simulink library "ddm"  (R2021b)
settings: Solver=VariableStepAuto  StartTime=0.0  StopTime=10.0  RelTol=1e-3
undefined symbols (not defined in the file or in its folder): ADDM_FrTMTqDev_X_Nm, ADDM_RrTMTqDev_X_Nm, ENUM_ADASACCSTA_ERROR, ENUM_ADASACCSTA_OFF, ENUM_ADASACCSTA_STANDBY, ENUM_ALLOWMOV_ALLOWREADY, ENUM_APS, ENUM_BRKSTA_ERROR, ENUM_BRKSTA_OFF, ENUM_BRKSTA_ON, ENUM_BRKSW_INVALID, ENUM_BRKSW_OFF, ENUM_BRKSW_ON, ENUM_CHGPREACTERRSTA_OBCPRE, ENUM_DCDCFAULTSTA_ANYFAULTLV1, ENUM_DCDCFAULTSTA_ANYFAULTLV2, ENUM_DRIVETRAIN_AWD, ENUM_DRIVETRAIN_FWD, ENUM_DRIVETRAIN_RWD, ENUM_EDUDRTSTA_NORMAL, ENUM_EPBSTA_APPLIED, ENUM_EPBSTA_RELEASED, ENUM_GEARACTUALPOSN_INVALID, ENUM_GEARACTUALPOSN_P, ENUM_HVBATTREADYPRE_READY, ENUM_MCUWARN_LV0, ENUM_MCUWARN_LV1, ENUM_MCUWARN_LV2, ENUM_MCUWARN_LV3, ENUM_MCUWARN_NOERROR, ENUM_OBCFAULTSTA_ANYFAULT, ENUM_PAS_R2F2, ENUM_PDFAULT_BATTPDFAIL, ENUM_PDFAULT_DCDCDISABLE, ENUM_PDFAULT_MCUDISABLE, ENUM_PDFAULT_MCUDISCHRG, ENUM_POWERSTA_OFF, ENUM_POWERSTA_ON, ENUM_POWERSTA_READY, ENUM_POWERSTA_STANDBY, ENUM_PRESSINDI_LOW, ENUM_PUFAULT_BATTUPFAIL, ENUM_PUFAULT_DCDCENABLEFAIL, ENUM_PUFAULT_PRECHRGCHKFAIL, ENUM_PUFAULT_SAFETYCHKFAIL, ENUM_PUSTATE_COMPLETED, ENUM_PWRSTASW_OFF, ENUM_PWRSTASW_OFFA, ENUM_PWRSTASW_OFFCHVCHRG, ENUM_PWRSTASW_OFFCLVCHRG, ENUM_PWRSTASW_ON, ENUM_PWRSTASW_ONHVCHRG, ENUM_PWRSTASW_READY, ENUM_PWRSTASW_STANDBY, ENUM_SHIFTCOMMAND_P, ENUM_SHIFTERERRSTA_PBUTTONFAILURE, ENUM_VEHMALFUNLV_2ND, ENUM_VEHMALFUNLV_3RD, ENUM_VEHMALFUNLV_4TH, ENUM_VEHMALFUNLV_NORMAL ... (+459)
libraries: hcu_lib x521, $bdroot x5, simulink x3
(part 15 of 25)

== system ddm/DDM/DDM/TQD/Shifter1_DDM ==
  note: Release Condition After Decision
  note: Diagnostics and Fault Handling
  note: Diagnostics and Fault Handling
  note: Release Condition After Decision
  note: Release Condition After Decision
  note: Diagnostics and Fault Handling
  note: Shifter1 Rolling Count Error (Shifter1CSErr)
  note: Shifter1 Rolling Count Error (Shifter1RCErr)
  note: Shifter1 Lost Comm (Shifter1NoCom)
  task_time_s : Inport
  VPMM_SysPwrSta_enum : Inport  Port=2
  No_CAN3_BUS_OFF : Inport  Port=3
  VDDM_Shifter1NoCom_flg : Inport  Port=4
  VDDM_Shifter1RCErr_flg : Inport  Port=5
  VDDM_Shifter1CSErr_flg : Inport  Port=6
  DTC_clear_request : Inport  Port=7
  VINP_ShifterHandleCmd_enum : Inport  Port=8
  Constant1 : Constant  Value=KDDM_Shifter1NoComDTC_cnt
  Constant10 : Constant  Value=KDDM_Shifter1CSErrDTC_cnt
  Constant{3,11,16..17,19,24,31,36,48} (9 alike) : Constant  Value=ENUM_PWRSTASW_OFF
  Constant12 : Constant  Value=FALSE
  Constant13 : Constant  Value=KDDM_Shifter1RCErrDTC_cnt
  Constant14 : Constant  Value=KDDM_Shifter1RCErrPassTO_s
  Constant15 : Constant  Value=ZERO_INT
  Constant18 : Constant  Value=KDDM_Shifter1RCErrDetTO_s
  Constant2 : Constant  Value=FALSE
  Constant20 : Constant  Value=KDDM_Shifter1NoComDTC_cnt
  Constant21 : Constant  Value=KDDM_Shifter1NoComPassTO_s
  Constant22 : Constant  Value=KDDM_Shifter1NoComDetTO_s
  Constant23 : Constant  Value=ENUM_SHIFTCOMMAND_P
  Constant25 : Constant  Value=KDDM_TQDDiagnosisOffSW_flg
  Constant26 : Constant  Value=ENUM_PWRSTASW_STANDBY
  Constant27 : Constant  Value=KDDM_Shifter1RCErrPassTO_s
  Constant32 : Constant  Value=FALSE
  Constant33 : Constant  Value=KDDM_Shifter1CSErrDTC_cnt
  Constant34 : Constant  Value=KDDM_Shifter1CSErrPassTO_s
  Constant35 : Constant  Value=KDDM_Shifter1CSErrDetTO_s
  Constant4 : Constant  Value=KDDM_Shifter1RCErrDTC_cnt
  Constant41 : Constant  Value=KDDM_Shifter1CSErrPassTO_s
  Constant42 : Constant  Value=ENUM_SHIFTCOMMAND_P
  Constant44 : Constant  Value=KDDM_TQDDiagnosisOffSW_flg
  Constant45 : Constant  Value=ZERO_INT
  Constant5 : Constant  Value=ENUM_SHIFTCOMMAND_P
  Constant6 : Constant  Value=ENUM_PWRSTASW_STANDBY
  Constant7 : Constant  Value=KDDM_TQDDiagnosisOffSW_flg
  Constant70 : Constant  Value=KDDM_Shifter1NoComPassTO_s
  Constant8 : Constant  Value=ZERO_INT
  Constant9 : Constant  Value=ENUM_PWRSTASW_STANDBY
  DTC_Couter1 : hcu_lib/Basic_Blocks/DTC_Couter
  DTC_Couter2 : hcu_lib/Basic_Blocks/DTC_Couter
  DTC_Couter4 : hcu_lib/Basic_Blocks/DTC_Couter
  DTC_Info : hcu_lib/Basic_Blocks/DTC_Info
  DTC_Info1 : hcu_lib/Basic_Blocks/DTC_Info
  DTC_Info2 : hcu_lib/Basic_Blocks/DTC_Info
  Equal{,1,3,10..11,16..19} (9 alike) : RelationalOperator  Operator===  OutDataTypeStr=boolean  RndMeth=Simplest
  Equal{2,4..6,13..14} (6 alike) : RelationalOperator  Operator=~=  OutDataTypeStr=boolean  RndMeth=Simplest
  Equal15 : RelationalOperator  OutDataTypeStr=boolean  RndMeth=Simplest
  Equal7 : RelationalOperator  OutDataTypeStr=boolean  RndMeth=Simplest
  Equal8 : RelationalOperator  OutDataTypeStr=boolean  RndMeth=Simplest
  Logical Operator : Logic  Operator=OR  Inputs=3  AllPortsSameDT=off  OutDataTypeStr=boolean
  Logical Operator1 : Logic  Operator=OR  Inputs=4  AllPortsSameDT=off  OutDataTypeStr=boolean
  Logical Operator10 : Logic  Inputs=3  AllPortsSameDT=off  OutDataTypeStr=boolean
  Logical Operator{2,5,8,11,50..51} (6 alike) : Logic  AllPortsSameDT=off  OutDataTypeStr=boolean
  Logical Operator{6,9,12,14,20,24,28,30,34,38} (10 alike) : Logic  Operator=NOT  AllPortsSameDT=off  OutDataTypeStr=boolean
  Logical Operator{4,22,26,36} (4 alike) : Logic  Inputs=4  AllPortsSameDT=off  OutDataTypeStr=boolean
  Logical Operator3 : Logic  Operator=OR  Inputs=4  AllPortsSameDT=off  OutDataTypeStr=boolean
  Logical Operator48 : Logic  Operator=OR  Inputs=4  AllPortsSameDT=off  OutDataTypeStr=boolean
  Logical Operator7 : Logic  Inputs=3  AllPortsSameDT=off  OutDataTypeStr=boolean
  Relational Operator1 : RelationalOperator  Operator=>  OutDataTypeStr=boolean  RndMeth=Simplest
  Relational Operator2 : RelationalOperator  Operator=>  OutDataTypeStr=boolean  RndMeth=Simplest
  Relational Operator3 : RelationalOperator  Operator=>  OutDataTypeStr=boolean  RndMeth=Simplest
  Switch1 : Switch  Criteria=u2 ~= 0
  Switch2 : Switch  Criteria=u2 ~= 0
  Switch6 : Switch  Criteria=u2 ~= 0
  Terminator : Terminator
  Terminator1 : Terminator
  Terminator2 : Terminator
  Test Detection Criteria1 : hcu_lib/Basic_Blocks/Test Detection Criteria
  Test Detection Criteria2 : hcu_lib/Basic_Blocks/Test Detection Criteria
  Test Detection Criteria3 : hcu_lib/Basic_Blocks/Test Detection Criteria
  Timer1 : hcu_lib/Basic_Blocks/Timer
  Timer2 : hcu_lib/Basic_Blocks/Timer
  Timer3 : hcu_lib/Basic_Blocks/Timer
  Unit Delay1 : UnitDelay  SampleTime=-1  HasFrameUpgradeWarning=on
  Unit Delay2 : UnitDelay  SampleTime=-1  HasFrameUpgradeWarning=on
  Unit Delay6 : UnitDelay  SampleTime=-1  HasFrameUpgradeWarning=on
  VDDM_Shifter1NoComDTC_raw32 : Outport
  VDDM_Shifter1RCErrDTC_raw32 : Outport  Port=2
  VDDM_Shifter1CSErrDTC_raw32 : Outport  Port=3
  VDDM_Shifter1NoComCFS_flg : Outport  Port=4
  VDDM_Shifter1RCErrCFS_flg : Outport  Port=5
  VDDM_Shifter1CSErrCFS_flg : Outport  Port=6
  VDDM_Shifter1Err_flg : Outport  Port=7
  wires:
  [VPMM_SysPwrSta_enum] -> Equal3/1
  DTC_Couter2/2 -> Relational Operator3/1  "VDDM_Shifter1CSErrDTC_cnt"
  Equal1/1 -> Logical Operator5/2
  [VINP_ShifterHandleCmd_enum] -> Equal1/1
  Logical Operator3/1 -> [VDDM_Shifter1CSErrCFSRls_flg]  "VDDM_Shifter1CSErrCFSRls_flg"
  Constant23/1 -> Equal1/2
  Constant24/1 -> Equal19/2
  Constant8/1 -> Relational Operator3/2
  Logical Operator5/1 -> Logical Operator3/3
  Equal19/1 -> Logical Operator8/1
  Unit Delay1/1 -> Equal19/1
  Constant25/1 -> Logical Operator3/4
  [VDDM_Shifter1CSErrPass_flg] -> Logical Operator5/1
  [VDDM_Shifter1CSErrDet_flg] -> DTC_Couter2/1
  DTC_Couter2/1 -> [VDDM_Shifter1CSErrCFS_flg]  "VDDM_Shifter1CSErrCFS_flg"
  Constant10/1 -> DTC_Couter2/3
  [VDDM_Shifter1CSErrCFSRls_flg] -> DTC_Couter2/2
  [DTC_clear_request] -> Logical Operator3/2
  Relational Operator3/1 -> Terminator2/1  "VDDM_Shifter1CSErrDFS_flg"
  Constant9/1 -> Equal3/2
  Logical Operator8/1 -> Logical Operator3/1
  [VPMM_SysPwrSta_enum] -> Unit Delay1/1
  Equal3/1 -> Logical Operator8/2
  Equal11/1 -> Logical Operator2/2
  DTC_Couter1/1 -> [VDDM_Shifter1RCErrCFS_flg]  "VDDM_Shifter1RCErrCFS_flg"
  [DTC_clear_request] -> Logical Operator1/2
  Logical Operator2/1 -> Logical Operator1/1
  [VPMM_SysPwrSta_enum] -> Unit Delay2/1
  Constant6/1 -> Equal11/2
  Relational Operator1/1 -> Terminator1/1  "VDDM_Shifter1RCErrDFS_flg"
  DTC_Couter1/2 -> Relational Operator1/1  "VDDM_Shifter1RCErrDTC_cnt"
  [VDDM_Shifter1RCErrCFSRls_flg] -> DTC_Couter1/2
  [VINP_ShifterHandleCmd_enum] -> Equal10/1
  Constant5/1 -> Equal10/2
  Equal10/1 -> Logical Operator11/2
  [VDDM_Shifter1RCErrPass_flg] -> Logical Operator11/1
  [VDDM_Shifter1RCErrDet_flg] -> DTC_Couter1/1
  Logical Operator11/1 -> Logical Operator1/3
  Constant15/1 -> Relational Operator1/2
  [VPMM_SysPwrSta_enum] -> Equal11/1
  Equal16/1 -> Logical Operator2/1
  Constant7/1 -> Logical Operator1/4
  Logical Operator1/1 -> [VDDM_Shifter1RCErrCFSRls_flg]  "VDDM_Shifter1RCErrCFSRls_flg"
  Constant16/1 -> Equal16/2
  Unit Delay2/1 -> Equal16/1
  Constant4/1 -> DTC_Couter1/3
  Equal/1 -> Logical Operator51/2
  Constant42/1 -> Equal/2
  [VINP_ShifterHandleCmd_enum] -> Equal/1
  VINP_ShifterHandleCmd_enum/1 -> [VINP_ShifterHandleCmd_enum]
  Constant48/1 -> Equal18/2
  Unit Delay6/1 -> Equal18/1
  DTC_Couter4/2 -> Relational Operator2/1  "VDDM_Shifter1NoComDTC_cnt"
  [DTC_clear_request] -> Logical Operator48/2
  Constant26/1 -> Equal17/2
  Logical Operator50/1 -> Logical Operator48/1
  [VPMM_SysPwrSta_enum] -> Unit Delay6/1
  Equal17/1 -> Logical Operator50/2
  Relational Operator2/1 -> Terminator/1  "VDDM_Shifter1NoComDFS_flg"
  Constant44/1 -> Logical Operator48/4
  [VPMM_SysPwrSta_enum] -> Equal17/1
  Equal18/1 -> Logical Operator50/1
  Constant1/1 -> DTC_Couter4/3
  [VDDM_Shifter1NoComDet_flg] -> DTC_Couter4/1
  [VDDM_Shifter1NoComPass_flg] -> Logical Operator51/1
  Constant45/1 -> Relational Operator2/2
  Logical Operator51/1 -> Logical Operator48/3
  Logical Operator48/1 -> [VDDM_Shifter1NoComCFSRls_flg]  "VDDM_Shifter1NoComCFSRls_flg"
  [VDDM_Shifter1NoComCFSRls_flg] -> DTC_Couter4/2
  DTC_Couter4/1 -> [VDDM_Shifter1NoComCFS_flg]  "VDDM_Shifter1NoComCFS_flg"
  [VDDM_Shifter1CSErrCFS_flg] -> VDDM_Shifter1CSErrCFS_flg/1
  [VDDM_Shifter1RCErrCFS_flg] -> VDDM_Shifter1RCErrCFS_flg/1
  [VDDM_Shifter1NoComCFS_flg] -> VDDM_Shifter1NoComCFS_flg/1
  Logical Operator28/1 -> Logical Operator36/4
  [VDDM_Shifter1NoComCFS_flg] -> Logical Operator28/1
  Logical Operator6/1 -> Logical Operator22/4
  [VDDM_Shifter1NoComCFS_flg] -> Logical Operator6/1
  VDDM_Shifter1CSErr_flg/1 -> [VDDM_Shifter1CSErr_flg]
  VDDM_Shifter1RCErr_flg/1 -> [VDDM_Shifter1RCErr_flg]
  Switch2/1 -> Test Detection Criteria3/1
  Switch1/1 -> Test Detection Criteria2/1
  Test Detection Criteria3/1 -> [VDDM_Shifter1CSErrDet_flg]  "VDDM_Shifter1CSErrDet_flg"
  [VDDM_Shifter1CSErr_flg] -> Logical Operator26/3
  [DTC_clear_request] -> DTC_Info2/4
  Logical Operator38/1 -> Logical Operator36/3
  Logical Operator26/1 -> Switch2/3
  [VDDM_Shifter1CSErrCFS_flg] -> DTC_Info2/3
  Constant32/1 -> Switch2/1
  [VDDM_Shifter1CSErrCFSRls_flg] -> Switch2/2
  Timer3/1 -> Equal15/1
  Constant41/1 -> Timer3/4
  [task_time_s] -> Test Detection Criteria3/2
  [task_time_s] -> Timer3/3
  [VDDM_Shifter1CSErrDet_flg] -> DTC_Info2/1
  [No_CAN3_BUS_OFF] -> Logical Operator26/2
  [VPMM_SysPwrSta_enum] -> Equal14/1
  DTC_Info2/1 -> VDDM_Shifter1CSErrDTC_raw32/1  "VDDM_Shifter1CSErrDTC_raw32"
  Equal13/1 -> Logical Operator36/1
  [No_CAN3_BUS_OFF] -> Logical Operator36/2
  [VDDM_Shifter1CSErrPass_flg] -> DTC_Info2/2
  Constant35/1 -> Test Detection Criteria3/4
  Constant31/1 -> Equal14/2
  Constant36/1 -> Equal13/2
  [VDDM_Shifter1CSErr_flg] -> Logical Operator38/1
  Constant34/1 -> Equal15/2
  [VDDM_Shifter1NoComCFS_flg] -> Logical Operator34/1
  Logical Operator36/1 -> Logical Operator30/1, Timer3/1
  Equal14/1 -> Logical Operator26/1
  Equal15/1 -> [VDDM_Shifter1CSErrPass_flg]  "VDDM_Shifter1CSErrPass_flg"
  Constant33/1 -> Test Detection Criteria3/3
  [VPMM_SysPwrSta_enum] -> Equal13/1
  Logical Operator30/1 -> Timer3/2
  Logical Operator34/1 -> Logical Operator26/4
  Test Detection Criteria2/1 -> [VDDM_Shifter1RCErrDet_flg]  "VDDM_Shifter1RCErrDet_flg"
  [VDDM_Shifter1RCErr_flg] -> Logical Operator4/3
  [DTC_clear_request] -> DTC_Info1/4
  Logical Operator24/1 -> Logical Operator22/3
  Logical Operator4/1 -> Switch1/3
  [VDDM_Shifter1RCErrCFS_flg] -> DTC_Info1/3
  Constant12/1 -> Switch1/1
  [VDDM_Shifter1RCErrCFSRls_flg] -> Switch1/2
  Timer1/1 -> Equal8/1
  Constant27/1 -> Timer1/4
  [task_time_s] -> Test Detection Criteria2/2
  [task_time_s] -> Timer1/3
  [VDDM_Shifter1RCErrDet_flg] -> DTC_Info1/1
  [No_CAN3_BUS_OFF] -> Logical Operator4/2
  [VPMM_SysPwrSta_enum] -> Equal5/1
  DTC_Info1/1 -> VDDM_Shifter1RCErrDTC_raw32/1  "VDDM_Shifter1RCErrDTC_raw32"
  Equal4/1 -> Logical Operator22/1
  [No_CAN3_BUS_OFF] -> Logical Operator22/2
  [VDDM_Shifter1RCErrPass_flg] -> DTC_Info1/2
  Constant18/1 -> Test Detection Criteria2/4
  Constant11/1 -> Equal5/2
  Constant19/1 -> Equal4/2
  [VDDM_Shifter1RCErr_flg] -> Logical Operator24/1
  Constant14/1 -> Equal8/2
  [VDDM_Shifter1NoComCFS_flg] -> Logical Operator20/1
  Logical Operator22/1 -> Logical Operator12/1, Timer1/1
  Equal5/1 -> Logical Operator4/1
  Equal8/1 -> [VDDM_Shifter1RCErrPass_flg]  "VDDM_Shifter1RCErrPass_flg"
  Constant13/1 -> Test Detection Criteria2/3
  [VPMM_SysPwrSta_enum] -> Equal4/1
  Logical Operator12/1 -> Timer1/2
  Logical Operator20/1 -> Logical Operator4/4
  Constant2/1 -> Switch6/1
  Logical Operator10/1 -> Switch6/3
  Switch6/1 -> Test Detection Criteria1/1
  [VDDM_Shifter1NoComCFSRls_flg] -> Switch6/2
  [DTC_clear_request] -> DTC_Info/4
  No_CAN3_BUS_OFF/1 -> [No_CAN3_BUS_OFF]
  [VDDM_Shifter1NoComDet_flg] -> DTC_Info/1
  DTC_clear_request/1 -> [DTC_clear_request]
  task_time_s/1 -> [task_time_s]
  [VDDM_Shifter1NoComPass_flg] -> DTC_Info/2
  DTC_Info/1 -> VDDM_Shifter1NoComDTC_raw32/1  "VDDM_Shifter1NoComDTC_raw32"
  [VDDM_Shifter1NoComCFS_flg] -> DTC_Info/3
  VPMM_SysPwrSta_enum/1 -> [VPMM_SysPwrSta_enum]
  VDDM_Shifter1NoCom_flg/1 -> [VDDM_Shifter1NoCom_flg]
  [VPMM_SysPwrSta_enum] -> Equal2/1
  [No_CAN3_BUS_OFF] -> Logical Operator7/2
  Constant3/1 -> Equal2/2
  Logical Operator9/1 -> Logical Operator7/3
  Equal2/1 -> Logical Operator7/1
  [VDDM_Shifter1NoCom_flg] -> Logical Operator9/1
  [VPMM_SysPwrSta_enum] -> Equal6/1
  [VDDM_Shifter1NoCom_flg] -> Logical Operator10/3
  Constant17/1 -> Equal6/2
  Equal6/1 -> Logical Operator10/1
  [No_CAN3_BUS_OFF] -> Logical Operator10/2
  [task_time_s] -> Timer2/3
  Constant21/1 -> Equal7/2
  [task_time_s] -> Test Detection Criteria1/2
  Constant70/1 -> Timer2/4
  Constant20/1 -> Test Detection Criteria1/3
  Test Detection Criteria1/1 -> [VDDM_Shifter1NoComDet_flg]  "VDDM_Shifter1NoComDet_flg"
  Equal7/1 -> [VDDM_Shifter1NoComPass_flg]  "VDDM_Shifter1NoComPass_flg"
  Timer2/1 -> Equal7/1
  Logical Operator7/1 -> Timer2/1, Logical Operator14/1
  Constant22/1 -> Test Detection Criteria1/4
  Logical Operator14/1 -> Timer2/2
  [VDDM_Shifter1NoComCFS_flg] -> Logical Operator/1
  [VDDM_Shifter1RCErrCFS_flg] -> Logical Operator/2
  [VDDM_Shifter1CSErrCFS_flg] -> Logical Operator/3
  Logical Operator/1 -> VDDM_Shifter1Err_flg/1  "VDDM_Shifter1Err_flg"

== system ddm/DDM/DDM/VMC_DDM/ACC Acceleration Command Error ==
  task_time_s : Inport
  VDDM_FCM1NoComCFS_flg : Inport  Port=2
  VDDM_FCM1RCErrCFS_flg : Inport  Port=3
  VDDM_FCM1CSErrCFS_flg : Inport  Port=4
  VVMC_ADASActive_flg : Inport  Port=5
  No_CAN6_BUS_OFF : Inport  Port=6
  VPMM_PowerSta_enum : Inport  Port=7
  VINP_ACCRequireAccel_mps2 : Inport  Port=8
  VINP_ADASACCSta_enum : Inport  Port=9
  DTC_clear_request : Inport  Port=10
  "ACC Acceleration Command Error " : Subsystem
  VDDM_ACCAccelCmdErrCFS_flg : Outport
  VDDM_ACCAccelCmdErrDetDTC_raw32 : Outport  Port=2
  wires:
  [VDDM_ACCAccelCmdErrDetDTC_raw32] -> VDDM_ACCAccelCmdErrDetDTC_raw32/1
  "ACC Acceleration Command Error "/2(VDDM_ACCAccelCmdErrDetDTC_raw32) -> [VDDM_ACCAccelCmdErrDetDTC_raw32]
  VINP_ADASACCSta_enum/1 -> [VINP_ADASACCSta_enum]
  [VINP_ADASACCSta_enum] -> "ACC Acceleration Command Error "/9(VINP_ADASACCSta_enum)
  [VVMC_ADASActive_flg] -> "ACC Acceleration Command Error "/5(VVMC_ADASActive_flg)
  VVMC_ADASActive_flg/1 -> [VVMC_ADASActive_flg]
  [task_time_s] -> "ACC Acceleration Command Error "/1(task_time_s)
  task_time_s/1 -> [task_time_s]  "task_time_s"
  [DTC_clear_request] -> "ACC Acceleration Command Error "/10(DTC_clear_request)
  [VINP_ACCRequireAccel_mps2] -> "ACC Acceleration Command Error "/8(VINP_ACCRequireAccel_mps2)
  [VPMM_PowerSta_enum] -> "ACC Acceleration Command Error "/7(VPMM_PowerSta_enum)
  [No_CAN6_BUS_OFF] -> "ACC Acceleration Command Error "/6(No_CAN6_BUS_OFF)
  [VDDM_FCM1CSErrCFS_flg] -> "ACC Acceleration Command Error "/4(VDDM_FCM1CSErrCFS_flg)
  [VDDM_FCM1RCErrCFS_flg] -> "ACC Acceleration Command Error "/3(VDDM_FCM1RCErrCFS_flg)
  [VDDM_FCM1NoComCFS_flg] -> "ACC Acceleration Command Error "/2(VDDM_FCM1NoComCFS_flg)
  VINP_ACCRequireAccel_mps2/1 -> [VINP_ACCRequireAccel_mps2]
  VDDM_FCM1NoComCFS_flg/1 -> [VDDM_FCM1NoComCFS_flg]
  No_CAN6_BUS_OFF/1 -> [No_CAN6_BUS_OFF]
  VPMM_PowerSta_enum/1 -> [VPMM_PowerSta_enum]
  DTC_clear_request/1 -> [DTC_clear_request]
  "ACC Acceleration Command Error "/1(VDDM_ACCAccelCmdErrCFS_flg) -> [VDDM_ACCAccelCmdErrCFS_flg]
  [VDDM_ACCAccelCmdErrCFS_flg] -> VDDM_ACCAccelCmdErrCFS_flg/1
  VDDM_FCM1RCErrCFS_flg/1 -> [VDDM_FCM1RCErrCFS_flg]
  VDDM_FCM1CSErrCFS_flg/1 -> [VDDM_FCM1CSErrCFS_flg]

== system ddm/DDM/DDM/VMC_DDM/BMS Signal Error  ==
  task_time_s : Inport
  VDDM_C3BMS6LCCFS_flg : Inport  Port=2
  VDDM_C3BMS6RCCFS_flg : Inport  Port=3
  VDDM_C3BMS6CSCFS_flg : Inport  Port=4
  No_CAN3_BUS_OFF : Inport  Port=5
  VPMM_PowerSta_enum : Inport  Port=6
  VINP_BMSWarn8_flg : Inport  Port=7
  VINP_BMSWarn7_flg : Inport  Port=8
  VINP_BMSWarn6_flg : Inport  Port=9
  VINP_BMSWarn5_flg : Inport  Port=10
  VINP_BMSWarn4_flg : Inport  Port=11
  VINP_BMSWarn3_flg : Inport  Port=12
  VINP_BMSWarn2_flg : Inport  Port=13
  VINP_BMSWarn1_flg : Inport  Port=14
  DTC_clear_request : Inport  Port=15
  "BMS Signal Error " : Subsystem
  VDDM_BMSSigErrCFS_flg : Outport
  VDDM_BMSSigErrDetDTC_raw32 : Outport  Port=2
  wires:
  [VDDM_BMSSigErrDetDTC_raw32] -> VDDM_BMSSigErrDetDTC_raw32/1
  "BMS Signal Error "/2(VDDM_BMSSigErrDetDTC_raw32) -> [VDDM_BMSSigErrDetDTC_raw32]
  [task_time_s] -> "BMS Signal Error "/1(task_time_s)
  task_time_s/1 -> [task_time_s]  "task_time_s"
  [VINP_BMSWarn8_flg] -> "BMS Signal Error "/15(VINP_BMSWarn8_flg)
  [VPMM_PowerSta_enum] -> "BMS Signal Error "/6(VPMM_PowerSta_enum)
  [No_CAN3_BUS_OFF] -> "BMS Signal Error "/5(No_CAN3_BUS_OFF)
  [VDDM_C3BMS6RCCFS_flg] -> "BMS Signal Error "/3(VDDM_C3BMS6RCCFS_flg)
  [VDDM_C3BMS6LCCFS_flg] -> "BMS Signal Error "/2(VDDM_C3BMS6LCCFS_flg)
  VINP_BMSWarn4_flg/1 -> [VINP_BMSWarn4_flg]
  VINP_BMSWarn6_flg/1 -> [VINP_BMSWarn6_flg]
  VINP_BMSWarn5_flg/1 -> [VINP_BMSWarn5_flg]
  VINP_BMSWarn7_flg/1 -> [VINP_BMSWarn7_flg]
  VINP_BMSWarn8_flg/1 -> [VINP_BMSWarn8_flg]
  VDDM_C3BMS6LCCFS_flg/1 -> [VDDM_C3BMS6LCCFS_flg]
  No_CAN3_BUS_OFF/1 -> [No_CAN3_BUS_OFF]
  VPMM_PowerSta_enum/1 -> [VPMM_PowerSta_enum]
  DTC_clear_request/1 -> [DTC_clear_request]
  "BMS Signal Error "/1(VDDM_BMSSigErrCFS_flg) -> [VDDM_BMSSigErrCFS_flg]
  [VDDM_BMSSigErrCFS_flg] -> VDDM_BMSSigErrCFS_flg/1
  VDDM_C3BMS6RCCFS_flg/1 -> [VDDM_C3BMS6RCCFS_flg]
  VDDM_C3BMS6CSCFS_flg/1 -> [VDDM_C3BMS6CSCFS_flg]
  [VDDM_C3BMS6CSCFS_flg] -> "BMS Signal Error "/4(VDDM_C3BMS6CSCFS_flg)
  [DTC_clear_request] -> "BMS Signal Error "/10(DTC_clear_request)
  [VINP_BMSWarn5_flg] -> "BMS Signal Error "/12(VINP_BMSWarn5_flg)
  [VINP_BMSWarn4_flg] -> "BMS Signal Error "/11(VINP_BMSWarn4_flg)
  [VINP_BMSWarn6_flg] -> "BMS Signal Error "/13(VINP_BMSWarn6_flg)
  [VINP_BMSWarn7_flg] -> "BMS Signal Error "/14(VINP_BMSWarn7_flg)
  [VINP_BMSWarn1_flg] -> "BMS Signal Error "/7(VINP_BMSWarn1_flg)
  [VINP_BMSWarn2_flg] -> "BMS Signal Error "/8(VINP_BMSWarn2_flg)
  [VINP_BMSWarn3_flg] -> "BMS Signal Error "/9(VINP_BMSWarn3_flg)
  VINP_BMSWarn3_flg/1 -> [VINP_BMSWarn3_flg]
  VINP_BMSWarn2_flg/1 -> [VINP_BMSWarn2_flg]
  VINP_BMSWarn1_flg/1 -> [VINP_BMSWarn1_flg]

== system ddm/DDM/DDM/VMC_DDM/CCU Signal Error ==
  task_time_s : Inport
  VDDM_C3CCU2LCCFS_flg : Inport  Port=2
  VDDM_C3CCU2RCCFS_flg : Inport  Port=3
  VDDM_C3CCU2CSCFS_flg : Inport  Port=4
  No_CAN3_BUS_OFF : Inport  Port=5
  VPMM_PowerSta_enum : Inport  Port=6
  VINP_DCDCFaultSta_enum : Inport  Port=7
  DTC_clear_request : Inport  Port=8
  "CCU Signal Error " : Subsystem
  VDDM_CCUSigErrCFS_flg : Outport
  VDDM_CCUSigErrDetDTC_raw32 : Outport  Port=2
  wires:
  [VDDM_CCUSigErrDetDTC_raw32] -> VDDM_CCUSigErrDetDTC_raw32/1
  "CCU Signal Error "/2(VDDM_CCUSigErrDetDTC_raw32) -> [VDDM_CCUSigErrDetDTC_raw32]
  [task_time_s] -> "CCU Signal Error "/1(task_time_s)
  task_time_s/1 -> [task_time_s]  "task_time_s"
  [DTC_clear_request] -> "CCU Signal Error "/8(DTC_clear_request)
  [VINP_DCDCFaultSta_enum] -> "CCU Signal Error "/7(VINP_DCDCFaultSta_enum)
  [VPMM_PowerSta_enum] -> "CCU Signal Error "/6(VPMM_PowerSta_enum)
  [No_CAN3_BUS_OFF] -> "CCU Signal Error "/5(No_CAN3_BUS_OFF)
  [VDDM_C3CCU2CSCFS_flg] -> "CCU Signal Error "/4(VDDM_C3CCU2CSCFS_flg)
  [VDDM_C3CCU2RCCFS_flg] -> "CCU Signal Error "/3(VDDM_C3CCU2RCCFS_flg)
  [VDDM_C3CCU2LCCFS_flg] -> "CCU Signal Error "/2(VDDM_C3CCU2LCCFS_flg)
  VINP_DCDCFaultSta_enum/1 -> [VINP_DCDCFaultSta_enum]
  VDDM_C3CCU2LCCFS_flg/1 -> [VDDM_C3CCU2LCCFS_flg]
  No_CAN3_BUS_OFF/1 -> [No_CAN3_BUS_OFF]
  VPMM_PowerSta_enum/1 -> [VPMM_PowerSta_enum]
  DTC_clear_request/1 -> [DTC_clear_request]
  "CCU Signal Error "/1(VDDM_CCUSigErrCFS_flg) -> [VDDM_CCUSigErrCFS_flg]
  [VDDM_CCUSigErrCFS_flg] -> VDDM_CCUSigErrCFS_flg/1
  VDDM_C3CCU2RCCFS_flg/1 -> [VDDM_C3CCU2RCCFS_flg]
  VDDM_C3CCU2CSCFS_flg/1 -> [VDDM_C3CCU2CSCFS_flg]

== system ddm/DDM/DDM/VMC_DDM/ESC Signal Error ==
  task_time_s : Inport
  No_CAN1_BUS_OFF : Inport  Port=2
  VPMM_PowerSta_enum : Inport  Port=3
  DTC_clear_request : Inport  Port=4
  VDDM_ESC1NoComCFS_flg : Inport  Port=5
  VDDM_ESC1RCErrCFS_flg : Inport  Port=6
  VDDM_ESC1CSErrCFS_flg : Inport  Port=7
  VDDM_ESC5NoComCFS_flg : Inport  Port=8
  VDDM_ESC5RCErrCFS_flg : Inport  Port=9
  VDDM_ESC5CSErrCFS_flg : Inport  Port=10
  VINP_HDDFailed_flg : Inport  Port=11
  VINP_EBDFailed_flg : Inport  Port=12
  VINP_ABSFailed_flg : Inport  Port=13
  VINP_TCSFailed_flg : Inport  Port=14
  VINP_ESCFailed_flg : Inport  Port=15
  VINP_HBBFailed_flg : Inport  Port=16
  VINP_PBAFailed_flg : Inport  Port=17
  VINP_HSAFailed_flg : Inport  Port=18
  VINP_AVHFailed_flg : Inport  Port=19
  VINP_MCPressureV_flg : Inport  Port=20
  VINP_BrkSwV_flg : Inport  Port=21
  VINP_BrkPedalPosSta_flg : Inport  Port=22
  VINP_LongAccelV_flg : Inport  Port=23
  VINP_LatAccelV_flg : Inport  Port=24
  VINP_YawRateV_flg : Inport  Port=25
  VINP_RFPulseCountV_flg : Inport  Port=26
  VINP_RRPulseCountV_flg : Inport  Port=27
  VINP_LFPulseCountV_flg : Inport  Port=28
  VINP_LRPulseCountV_flg : Inport  Port=29
  VINP_LRRawWhlSpeedV_flg : Inport  Port=30
  VINP_RRRawWhlSpeedV_flg : Inport  Port=31
  VINP_LFRawWhlSpeedV_flg : Inport  Port=32
  VINP_RFRawWhlSpeedV_flg : Inport  Port=33
  "ESC Signal Error " : Subsystem
  VDDM_ESCSigErrCFS_flg : Outport
  VDDM_ESCSigErrDetDTC_raw32 : Outport  Port=2
  VDDM_ESC1SigErr_flg : Outport  Port=3
  VDDM_ESC5SigErr_flg : Outport  Port=4
  wires:
  [VDDM_ESC5SigErr_flg] -> VDDM_ESC5SigErr_flg/1
  [VDDM_ESC1SigErr_flg] -> VDDM_ESC1SigErr_flg/1
  "ESC Signal Error "/4(VDDM_ESC5SigErr_flg) -> [VDDM_ESC5SigErr_flg]
  "ESC Signal Error "/3(VDDM_ESC1SigErr_flg) -> [VDDM_ESC1SigErr_flg]
  [VINP_RFRawWhlSpeedV_flg] -> "ESC Signal Error "/33(VINP_RFRawWhlSpeedV_flg)
  [VINP_LFRawWhlSpeedV_flg] -> "ESC Signal Error "/32(VINP_LFRawWhlSpeedV_flg)
  [VINP_RRRawWhlSpeedV_flg] -> "ESC Signal Error "/31(VINP_RRRawWhlSpeedV_flg)
  [VINP_LRRawWhlSpeedV_flg] -> "ESC Signal Error "/30(VINP_LRRawWhlSpeedV_flg)
  [VINP_LRPulseCountV_flg] -> "ESC Signal Error "/29(VINP_LRPulseCountV_flg)
  [VINP_LFPulseCountV_flg] -> "ESC Signal Error "/28(VINP_LFPulseCountV_flg)
  [VINP_RRPulseCountV_flg] -> "ESC Signal Error "/27(VINP_RRPulseCountV_flg)
  [VINP_RFPulseCountV_flg] -> "ESC Signal Error "/26(VINP_RFPulseCountV_flg)
  VINP_RFRawWhlSpeedV_flg/1 -> [VINP_RFRawWhlSpeedV_flg]
  VINP_RRRawWhlSpeedV_flg/1 -> [VINP_RRRawWhlSpeedV_flg]
  VINP_LFRawWhlSpeedV_flg/1 -> [VINP_LFRawWhlSpeedV_flg]
  VINP_LRRawWhlSpeedV_flg/1 -> [VINP_LRRawWhlSpeedV_flg]
  VINP_LRPulseCountV_flg/1 -> [VINP_LRPulseCountV_flg]
  VINP_LFPulseCountV_flg/1 -> [VINP_LFPulseCountV_flg]
  VINP_RRPulseCountV_flg/1 -> [VINP_RRPulseCountV_flg]
  VINP_RFPulseCountV_flg/1 -> [VINP_RFPulseCountV_flg]
  [VDDM_ESCSigErrCFS_flg] -> VDDM_ESCSigErrCFS_flg/1
  [VINP_YawRateV_flg] -> "ESC Signal Error "/25(VINP_YawRateV_flg)
  [VINP_LatAccelV_flg] -> "ESC Signal Error "/24(VINP_LatAccelV_flg)
  [VINP_LongAccelV_flg] -> "ESC Signal Error "/23(VINP_LongAccelV_flg)
  [VINP_BrkPedalPosSta_flg] -> "ESC Signal Error "/22(VINP_BrkPedalPosSta_flg)
  [VINP_BrkSwV_flg] -> "ESC Signal Error "/21(VINP_BrkSwV_flg)
  [VINP_MCPressureV_flg] -> "ESC Signal Error "/20(VINP_MCPressureV_flg)
  [VINP_AVHFailed_flg] -> "ESC Signal Error "/19(VINP_AVHFailed_flg)
  [VINP_HSAFailed_flg] -> "ESC Signal Error "/18(VINP_HSAFailed_flg)
  [VINP_PBAFailed_flg] -> "ESC Signal Error "/17(VINP_PBAFailed_flg)
  [VINP_HBBFailed_flg] -> "ESC Signal Error "/16(VINP_HBBFailed_flg)
  [VINP_ESCFailed_flg] -> "ESC Signal Error "/15(VINP_ESCFailed_flg)
  [VINP_TCSFailed_flg] -> "ESC Signal Error "/14(VINP_TCSFailed_flg)
  [VINP_ABSFailed_flg] -> "ESC Signal Error "/13(VINP_ABSFailed_flg)
  [VINP_EBDFailed_flg] -> "ESC Signal Error "/12(VINP_EBDFailed_flg)
  [VINP_HDDFailed_flg] -> "ESC Signal Error "/11(VINP_HDDFailed_flg)
  VINP_YawRateV_flg/1 -> [VINP_YawRateV_flg]
  VINP_LatAccelV_flg/1 -> [VINP_LatAccelV_flg]
  VINP_LongAccelV_flg/1 -> [VINP_LongAccelV_flg]
  VINP_BrkPedalPosSta_flg/1 -> [VINP_BrkPedalPosSta_flg]
  VINP_BrkSwV_flg/1 -> [VINP_BrkSwV_flg]
  VINP_MCPressureV_flg/1 -> [VINP_MCPressureV_flg]
  VINP_AVHFailed_flg/1 -> [VINP_AVHFailed_flg]
  VINP_HSAFailed_flg/1 -> [VINP_HSAFailed_flg]
  VINP_PBAFailed_flg/1 -> [VINP_PBAFailed_flg]
  VINP_HBBFailed_flg/1 -> [VINP_HBBFailed_flg]
  VINP_ESCFailed_flg/1 -> [VINP_ESCFailed_flg]
  VINP_TCSFailed_flg/1 -> [VINP_TCSFailed_flg]
  VINP_ABSFailed_flg/1 -> [VINP_ABSFailed_flg]
  VINP_EBDFailed_flg/1 -> [VINP_EBDFailed_flg]
  VINP_HDDFailed_flg/1 -> [VINP_HDDFailed_flg]
  [VDDM_ESC5CSErrCFS_flg] -> "ESC Signal Error "/10(VDDM_ESC5CSErrCFS_flg)
  [VDDM_ESC5RCErrCFS_flg] -> "ESC Signal Error "/9(VDDM_ESC5RCErrCFS_flg)
  [VDDM_ESC5NoComCFS_flg] -> "ESC Signal Error "/8(VDDM_ESC5NoComCFS_flg)
  VDDM_ESC5NoComCFS_flg/1 -> [VDDM_ESC5NoComCFS_flg]
  VDDM_ESC5RCErrCFS_flg/1 -> [VDDM_ESC5RCErrCFS_flg]
  VDDM_ESC5CSErrCFS_flg/1 -> [VDDM_ESC5CSErrCFS_flg]
  "ESC Signal Error "/1(VDDM_ESCSigErrCFS_flg) -> [VDDM_ESCSigErrCFS_flg]
  DTC_clear_request/1 -> [DTC_clear_request]
  VPMM_PowerSta_enum/1 -> [VPMM_PowerSta_enum]
  No_CAN1_BUS_OFF/1 -> [No_CAN1_BUS_OFF]
  [No_CAN1_BUS_OFF] -> "ESC Signal Error "/2(No_CAN1_BUS_OFF)
  [VPMM_PowerSta_enum] -> "ESC Signal Error "/3(VPMM_PowerSta_enum)
  [DTC_clear_request] -> "ESC Signal Error "/4(DTC_clear_request)
  task_time_s/1 -> [task_time_s]  "task_time_s"
  [task_time_s] -> "ESC Signal Error "/1(task_time_s)
  "ESC Signal Error "/2(VDDM_ESCSigErrDetDTC_raw32) -> [VDDM_ESCSigErrDetDTC_raw32]
  [VDDM_ESCSigErrDetDTC_raw32] -> VDDM_ESCSigErrDetDTC_raw32/1
  VDDM_ESC1NoComCFS_flg/1 -> [VDDM_ESC1NoComCFS_flg]
  VDDM_ESC1RCErrCFS_flg/1 -> [VDDM_ESC1RCErrCFS_flg]
  VDDM_ESC1CSErrCFS_flg/1 -> [VDDM_ESC1CSErrCFS_flg]
  [VDDM_ESC1NoComCFS_flg] -> "ESC Signal Error "/5(VDDM_ESC1NoComCFS_flg)
  [VDDM_ESC1RCErrCFS_flg] -> "ESC Signal Error "/6(VDDM_ESC1RCErrCFS_flg)
  [VDDM_ESC1CSErrCFS_flg] -> "ESC Signal Error "/7(VDDM_ESC1CSErrCFS_flg)

== system ddm/DDM/DDM/VMC_DDM/Enabled Subsystem ==
  task_time_s : Inport
  VPMM_PowerSta_enum : Inport  Port=2
  VDDM_EPS1NoCom_flg : Inport  Port=3
  No_CAN1_BUS_OFF : Inport  Port=4
  DTC_clear_request : Inport  Port=5
  VTQD_GearActualPosn_enum : Inport  Port=6
  VDDM_EPSRCErr_flg : Inport  Port=7
  VDDM_EPSCSErr_flg : Inport  Port=8
  VINP_SASV_flg : Inport  Port=9
  EPS1 Checksum Error : Subsystem
  EPS1 Lost Comm : Subsystem
  "EPS1 Rolling Count Error " : Subsystem
  EPS1 Signal Error : Subsystem
  VDDM_EPS1NoComCFS_flg : Outport
  VDDM_EPS1NoComDTC_raw32 : Outport  Port=2
  VDDM_EPS1RCErrCFS_flg : Outport  Port=3
  VDDM_EPS1RCErrDTC_raw32 : Outport  Port=4
  VDDM_EPS1CSErrCFS_flg : Outport  Port=5
  VDDM_EPS1CSErrDTC_raw32 : Outport  Port=6
  VDDM_EPSSigErrCFS_flg : Outport  Port=7
  VDDM_EPSSigErrDTC_raw32 : Outport  Port=8
  wires:
  [task_time_s] -> EPS1 Lost Comm/1(task_time_s)
  [VPMM_PowerSta_enum] -> EPS1 Lost Comm/2(VPMM_PowerSta_enum)
  [VDDM_EPS1NoCom_flg] -> EPS1 Lost Comm/3(VDDM_EPS1NoCom_flg)
  [No_CAN1_BUS_OFF] -> EPS1 Lost Comm/4(No_CAN1_BUS_OFF)
  [DTC_clear_request] -> EPS1 Lost Comm/5(DTC_clear_request)
  [VTQD_GearActualPosn_enum] -> EPS1 Lost Comm/6(VTQD_GearActualPosn_enum)
  EPS1 Lost Comm/2(VDDM_EPS1NoComDTC_raw32) -> [VDDM_EPS1NoComDTC_raw32]
  EPS1 Lost Comm/1(VDDM_EPS1NoComCFS_flg) -> [VDDM_EPS1NoComCFS_flg]
  task_time_s/1 -> [task_time_s]
  VPMM_PowerSta_enum/1 -> [VPMM_PowerSta_enum]
  VDDM_EPS1NoCom_flg/1 -> [VDDM_EPS1NoCom_flg]
  No_CAN1_BUS_OFF/1 -> [No_CAN1_BUS_OFF]
  DTC_clear_request/1 -> [DTC_clear_request]
  VTQD_GearActualPosn_enum/1 -> [VTQD_GearActualPosn_enum]
  [VDDM_EPS1NoComCFS_flg] -> VDDM_EPS1NoComCFS_flg/1
  [VDDM_EPS1NoComDTC_raw32] -> VDDM_EPS1NoComDTC_raw32/1
  [task_time_s] -> "EPS1 Rolling Count Error "/1(task_time_s)
  [VDDM_EPSRCErr_flg] -> "EPS1 Rolling Count Error "/2(VDDM_EPSRCErr_flg)
  VDDM_EPSRCErr_flg/1 -> [VDDM_EPSRCErr_flg]
  [No_CAN1_BUS_OFF] -> "EPS1 Rolling Count Error "/3(No_CAN1_BUS_OFF)
  [VDDM_EPS1NoComCFS_flg] -> "EPS1 Rolling Count Error "/4(VDDM_EPS1NoComCFS_flg)
  [VPMM_PowerSta_enum] -> "EPS1 Rolling Count Error "/5(VPMM_PowerSta_enum)
  [DTC_clear_request] -> "EPS1 Rolling Count Error "/6(DTC_clear_request)
  [VTQD_GearActualPosn_enum] -> "EPS1 Rolling Count Error "/7(VTQD_GearActualPosn_enum)
  "EPS1 Rolling Count Error "/1(VDDM_EPS1RCErrCFS_flg) -> [VDDM_EPS1RCErrCFS_flg]
  "EPS1 Rolling Count Error "/2(VDDM_EPS1RCErrDTC_raw32) -> [VDDM_EPS1RCErrDTC_raw32]
  [VDDM_EPS1RCErrCFS_flg] -> VDDM_EPS1RCErrCFS_flg/1
  [VDDM_EPS1RCErrDTC_raw32] -> VDDM_EPS1RCErrDTC_raw32/1
  [task_time_s] -> EPS1 Checksum Error/1(task_time_s)
  [VDDM_EPSCSErr_flg] -> EPS1 Checksum Error/2(VDDM_EPSCSErr_flg)
  [No_CAN1_BUS_OFF] -> EPS1 Checksum Error/3(No_CAN1_BUS_OFF)
  [VDDM_EPS1NoComCFS_flg] -> EPS1 Checksum Error/4(VDDM_EPS1NoComCFS_flg)
  [VPMM_PowerSta_enum] -> EPS1 Checksum Error/5(VPMM_PowerSta_enum)
  [DTC_clear_request] -> EPS1 Checksum Error/6(DTC_clear_request)
  [VTQD_GearActualPosn_enum] -> EPS1 Checksum Error/7(VTQD_GearActualPosn_enum)
  VDDM_EPSCSErr_flg/1 -> [VDDM_EPSCSErr_flg]
  EPS1 Checksum Error/1(VDDM_EPS1CSErrCFS_flg) -> [VDDM_EPS1CSErrCFS_flg]
  EPS1 Checksum Error/2(VDDM_EPS1CSErrDTC_raw32) -> [VDDM_EPS1CSErrDTC_raw32]
  [VDDM_EPS1CSErrCFS_flg] -> VDDM_EPS1CSErrCFS_flg/1
  [VDDM_EPS1CSErrDTC_raw32] -> VDDM_EPS1CSErrDTC_raw32/1
  [task_time_s] -> EPS1 Signal Error/1(task_time_s)
  [VINP_SASV_flg] -> EPS1 Signal Error/2(VINP_SASV_flg)
  [No_CAN1_BUS_OFF] -> EPS1 Signal Error/3(No_CAN1_BUS_OFF)
  [VDDM_EPS1NoComCFS_flg] -> EPS1 Signal Error/4(VDDM_EPS1NoComCFS_flg)
  [VPMM_PowerSta_enum] -> EPS1 Signal Error/5(VPMM_PowerSta_enum)
  [DTC_clear_request] -> EPS1 Signal Error/6(DTC_clear_request)
  [VDDM_EPS1RCErrCFS_flg] -> EPS1 Signal Error/7(VDDM_EPS1RCErrCFS_flg)
  [VDDM_EPS1CSErrCFS_flg] -> EPS1 Signal Error/8(VDDM_EPS1CSErrCFS_flg)
  [VTQD_GearActualPosn_enum] -> EPS1 Signal Error/9(VTQD_GearActualPosn_enum)
  EPS1 Signal Error/1(VDDM_EPSSigErrCFS_flg) -> [VDDM_EPSSigErrCFS_flg]
  EPS1 Signal Error/2(VDDM_EPSSigErrDTC_raw32) -> [VDDM_EPSSigErrDTC_raw32]
  [VDDM_EPSSigErrCFS_flg] -> VDDM_EPSSigErrCFS_flg/1
  [VDDM_EPSSigErrDTC_raw32] -> VDDM_EPSSigErrDTC_raw32/1
  VINP_SASV_flg/1 -> [VINP_SASV_flg]

== system ddm/DDM/DDM/VMC_DDM/FCM1 ==
  task_time_s : Inport
  VDDM_FCM1NoCom_flg : Inport  Port=2
  VDDM_FCM1RCErr_flg : Inport  Port=3
  VDDM_FCM1CSErr_flg : Inport  Port=4
  No_CAN6_BUS_OFF : Inport  Port=5
  VPMM_PowerSta_enum : Inport  Port=6
  DTC_clear_request : Inport  Port=7
  "FCM1 Checksum Error " : Subsystem  AncestorBlock=ddm/DDM/DDM/VMC_DDM/FCM2/FCM2 Checksum Error
  FCM1 Lost Com : Subsystem  AncestorBlock=ddm/DDM/DDM/VMC_DDM/FCM2/FCM2 Lost Com
  "FCM1 Rolling Count Error " : Subsystem  AncestorBlock=ddm/DDM/DDM/VMC_DDM/FCM2/FCM2 Rolling Count Error
  VDDM_FCM1NoComCFS_flg : Outport
  VDDM_FCM1RCErrCFS_flg : Outport  Port=2
  VDDM_FCM1CSErrCFS_flg : Outport  Port=3
  VDDM_FCM1NoComDTC_raw32 : Outport  Port=4
  VDDM_FCM1RCErrDTC_raw32 : Outport  Port=5
  VDDM_FCM1CSErrDTC_raw32 : Outport  Port=6
  wires:
  [VDDM_FCM1CSErrDTC_raw32] -> VDDM_FCM1CSErrDTC_raw32/1
  [VDDM_FCM1RCErrDTC_raw32] -> VDDM_FCM1RCErrDTC_raw32/1
  [VDDM_FCM1NoComDTC_raw32] -> VDDM_FCM1NoComDTC_raw32/1
  "FCM1 Checksum Error "/2(VDDM_FCM1CSErrDTC_raw32) -> [VDDM_FCM1CSErrDTC_raw32]
  "FCM1 Rolling Count Error "/2(VDDM_FCM1RCErrDTC_raw32) -> [VDDM_FCM1RCErrDTC_raw32]
  FCM1 Lost Com/2(VDDM_FCM1NoComDTC_raw32) -> [VDDM_FCM1NoComDTC_raw32]
  "FCM1 Checksum Error "/1(VDDM_FCM1CSErrCFS_flg) -> [VDDM_FCM1CSErrCFS_flg]
  [VDDM_FCM1NoComCFS_flg] -> "FCM1 Checksum Error "/4(VDDM_FCM1NoComCFS_flg)
  [VDDM_FCM1CSErr_flg] -> "FCM1 Checksum Error "/2(VDDM_FCM1CSErr_flg)
  [No_CAN6_BUS_OFF] -> "FCM1 Checksum Error "/3(No_CAN6_BUS_OFF)
  [VPMM_PowerSta_enum] -> "FCM1 Checksum Error "/5(VPMM_PowerSta_enum)
  [DTC_clear_request] -> "FCM1 Checksum Error "/6(DTC_clear_request)
  [task_time_s] -> "FCM1 Checksum Error "/1(task_time_s)
  [task_time_s] -> "FCM1 Rolling Count Error "/1(task_time_s)
  task_time_s/1 -> [task_time_s]  "task_time_s"
  [task_time_s] -> FCM1 Lost Com/1(task_time_s)
  VDDM_FCM1CSErr_flg/1 -> [VDDM_FCM1CSErr_flg]
  VDDM_FCM1RCErr_flg/1 -> [VDDM_FCM1RCErr_flg]
  [VDDM_FCM1RCErrCFS_flg] -> VDDM_FCM1RCErrCFS_flg/1
  [VDDM_FCM1CSErrCFS_flg] -> VDDM_FCM1CSErrCFS_flg/1
  [VDDM_FCM1NoComCFS_flg] -> VDDM_FCM1NoComCFS_flg/1
  "FCM1 Rolling Count Error "/1(VDDM_FCM1RCErrCFS_flg) -> [VDDM_FCM1RCErrCFS_flg]
  [DTC_clear_request] -> "FCM1 Rolling Count Error "/6(DTC_clear_request)
  [VPMM_PowerSta_enum] -> "FCM1 Rolling Count Error "/5(VPMM_PowerSta_enum)
  [No_CAN6_BUS_OFF] -> "FCM1 Rolling Count Error "/3(No_CAN6_BUS_OFF)
  [VDDM_FCM1RCErr_flg] -> "FCM1 Rolling Count Error "/2(VDDM_FCM1RCErr_flg)
  [VDDM_FCM1NoComCFS_flg] -> "FCM1 Rolling Count Error "/4(VDDM_FCM1NoComCFS_flg)
  FCM1 Lost Com/1(VDDM_FCM1NoComCFS_flg) -> [VDDM_FCM1NoComCFS_flg]
  [DTC_clear_request] -> FCM1 Lost Com/5(DTC_clear_request)
  [VPMM_PowerSta_enum] -> FCM1 Lost Com/4(VPMM_PowerSta_enum)
  [No_CAN6_BUS_OFF] -> FCM1 Lost Com/3(No_CAN6_BUS_OFF)
  DTC_clear_request/1 -> [DTC_clear_request]
  VPMM_PowerSta_enum/1 -> [VPMM_PowerSta_enum]
  No_CAN6_BUS_OFF/1 -> [No_CAN6_BUS_OFF]
  [VDDM_FCM1NoCom_flg] -> FCM1 Lost Com/2(VDDM_FCM1NoCom_flg)
  VDDM_FCM1NoCom_flg/1 -> [VDDM_FCM1NoCom_flg]

== system ddm/DDM/DDM/VMC_DDM/FCMACC Signal Error ==
  task_time_s : Inport
  VDDM_FCM1NoComCFS_flg : Inport  Port=2
  VDDM_FCM1RCErrCFS_flg : Inport  Port=3
  VDDM_FCM1CSErrCFS_flg : Inport  Port=4
  No_CAN6_BUS_OFF : Inport  Port=5
  VPMM_PowerSta_enum : Inport  Port=6
  VINP_ADASACCSta_enum : Inport  Port=7
  DTC_clear_request : Inport  Port=8
  VTQD_ExternalTqAllow_flg : Inport  Port=9
  VTQD_ExtDoorAllow_flg : Inport  Port=10
  "FCMACC Signal Error " : Subsystem
  VDDM_FCMACCSigErrCFS_flg : Outport
  VDDM_FCMACCSigErrDetDTC_raw32 : Outport  Port=2
  wires:
  VDDM_FCM1CSErrCFS_flg/1 -> [VDDM_FCM1CSErrCFS_flg]
  [VDDM_FCMACCSigErrCFS_flg] -> VDDM_FCMACCSigErrCFS_flg/1
  "FCMACC Signal Error "/1(VDDM_FCMACCSigErrCFS_flg) -> [VDDM_FCMACCSigErrCFS_flg]
  DTC_clear_request/1 -> [DTC_clear_request]
  VPMM_PowerSta_enum/1 -> [VPMM_PowerSta_enum]
  No_CAN6_BUS_OFF/1 -> [No_CAN6_BUS_OFF]
  VDDM_FCM1NoComCFS_flg/1 -> [VDDM_FCM1NoComCFS_flg]
  [No_CAN6_BUS_OFF] -> "FCMACC Signal Error "/5(No_CAN6_BUS_OFF)
  [VPMM_PowerSta_enum] -> "FCMACC Signal Error "/6(VPMM_PowerSta_enum)
  [DTC_clear_request] -> "FCMACC Signal Error "/8(DTC_clear_request)
  task_time_s/1 -> [task_time_s]  "task_time_s"
  [task_time_s] -> "FCMACC Signal Error "/1(task_time_s)
  [VDDM_FCM1NoComCFS_flg] -> "FCMACC Signal Error "/2(VDDM_FCM1NoComCFS_flg)
  [VDDM_FCM1CSErrCFS_flg] -> "FCMACC Signal Error "/4(VDDM_FCM1CSErrCFS_flg)
  VINP_ADASACCSta_enum/1 -> [VINP_ADASACCSta_enum]
  [VINP_ADASACCSta_enum] -> "FCMACC Signal Error "/7(VINP_ADASACCSta_enum)
  "FCMACC Signal Error "/2(VDDM_FCMACCSigErrDetDTC_raw32) -> [VDDM_FCMACCSigErrDetDTC_raw32]
  [VDDM_FCMACCSigErrDetDTC_raw32] -> VDDM_FCMACCSigErrDetDTC_raw32/1
  VTQD_ExternalTqAllow_flg/1 -> [VTQD_ExternalTqAllow_flg]
  VTQD_ExtDoorAllow_flg/1 -> [VTQD_ExtDoorAllow_flg]
  [VTQD_ExternalTqAllow_flg] -> "FCMACC Signal Error "/9(VTQD_ExternalTqAllow_flg)
  [VTQD_ExtDoorAllow_flg] -> "FCMACC Signal Error "/10(VTQD_ExtDoorAllow_flg)
  VDDM_FCM1RCErrCFS_flg/1 -> [VDDM_FCM1RCErrCFS_flg]
  [VDDM_FCM1RCErrCFS_flg] -> "FCMACC Signal Error "/3(VDDM_FCM1RCErrCFS_flg)

== system ddm/DDM/DDM/VMC_DDM/MCU_Fr Signal Error ==
  task_time_s : Inport
  VDDM_MCUNF1NoComCFS_flg : Inport  Port=2
  VDDM_MCUNF1RCErrCFS_flg : Inport  Port=3
  VDDM_MCUNF1CSErrCFS_flg : Inport  Port=4
  No_CAN3_BUS_OFF : Inport  Port=5
  VPMM_PowerSta_enum : Inport  Port=6
  VINP_MCUWarnFNidec_enum : Inport  Port=7
  DTC_clear_request : Inport  Port=8
  VPMM_DrivetrainSelect_enum : Inport  Port=9
  "MCU_Fr Signal Error " : Subsystem
  VDDM_FrMCUSigErrCFS_flg : Outport
  VDDM_FrMCUSigErrDetDTC_raw32 : Outport  Port=2
  wires:
  [VPMM_DrivetrainSelect_enum] -> "MCU_Fr Signal Error "/9(VPMM_DrivetrainSelect_enum)
  VPMM_DrivetrainSelect_enum/1 -> [VPMM_DrivetrainSelect_enum]
  [VDDM_FrMCUSigErrDetDTC_raw32] -> VDDM_FrMCUSigErrDetDTC_raw32/1
  "MCU_Fr Signal Error "/2(VDDM_FrMCUSigErrDetDTC_raw32) -> [VDDM_FrMCUSigErrDetDTC_raw32]
  [task_time_s] -> "MCU_Fr Signal Error "/1(task_time_s)
  task_time_s/1 -> [task_time_s]  "task_time_s"
  [DTC_clear_request] -> "MCU_Fr Signal Error "/8(DTC_clear_request)
  [VINP_MCUWarnFNidec_enum] -> "MCU_Fr Signal Error "/7(VINP_MCUWarnFNidec_enum)
  [VPMM_PowerSta_enum] -> "MCU_Fr Signal Error "/6(VPMM_PowerSta_enum)
  [No_CAN3_BUS_OFF] -> "MCU_Fr Signal Error "/5(No_CAN3_BUS_OFF)
  [VDDM_MCUNF1CSErrCFS_flg] -> "MCU_Fr Signal Error "/4(VDDM_MCUNF1CSErrCFS_flg)
  [VDDM_MCUNF1RCErrCFS_flg] -> "MCU_Fr Signal Error "/3(VDDM_MCUNF1RCErrCFS_flg)
  [VDDM_MCUNF1NoComCFS_flg] -> "MCU_Fr Signal Error "/2(VDDM_MCUNF1NoComCFS_flg)
  VINP_MCUWarnFNidec_enum/1 -> [VINP_MCUWarnFNidec_enum]
  VDDM_MCUNF1NoComCFS_flg/1 -> [VDDM_MCUNF1NoComCFS_flg]
  No_CAN3_BUS_OFF/1 -> [No_CAN3_BUS_OFF]
  VPMM_PowerSta_enum/1 -> [VPMM_PowerSta_enum]
  DTC_clear_request/1 -> [DTC_clear_request]
  "MCU_Fr Signal Error "/1(VDDM_FrMCUSigErrCFS_flg) -> [VDDM_FrMCUSigErrCFS_flg]
  [VDDM_FrMCUSigErrCFS_flg] -> VDDM_FrMCUSigErrCFS_flg/1
  VDDM_MCUNF1RCErrCFS_flg/1 -> [VDDM_MCUNF1RCErrCFS_flg]
  VDDM_MCUNF1CSErrCFS_flg/1 -> [VDDM_MCUNF1CSErrCFS_flg]

== system ddm/DDM/DDM/VMC_DDM/MCU_Rr Signal Error ==
  task_time_s : Inport
  VDDM_MCUNR1NoComCFS_flg : Inport  Port=2
  VDDM_MCUNR1RCErrCFS_flg : Inport  Port=3
  VDDM_MCUNR1CSErrCFS_flg : Inport  Port=4
  No_CAN3_BUS_OFF : Inport  Port=5
  VPMM_PowerSta_enum : Inport  Port=6
  VINP_MCUWarnRNidec_enum : Inport  Port=7
  DTC_clear_request : Inport  Port=8
  VPMM_DrivetrainSelect_enum : Inport  Port=9
  "MCU_Rr Signal Error " : Subsystem
  VDDM_RrMCUSigErrCFS_flg : Outport
  VDDM_RrMCUSigErrDetDTC_raw32 : Outport  Port=2
  wires:
  [VPMM_DrivetrainSelect_enum] -> "MCU_Rr Signal Error "/9(VPMM_DrivetrainSelect_enum)
  VPMM_DrivetrainSelect_enum/1 -> [VPMM_DrivetrainSelect_enum]
  [VDDM_RrMCUSigErrDetDTC_raw32] -> VDDM_RrMCUSigErrDetDTC_raw32/1
  "MCU_Rr Signal Error "/2(VDDM_RrMCUSigErrDetDTC_raw32) -> [VDDM_RrMCUSigErrDetDTC_raw32]
  [task_time_s] -> "MCU_Rr Signal Error "/1(task_time_s)
  task_time_s/1 -> [task_time_s]  "task_time_s"
  [DTC_clear_request] -> "MCU_Rr Signal Error "/8(DTC_clear_request)
  [VINP_MCUWarnRNidec_enum] -> "MCU_Rr Signal Error "/7(VINP_MCUWarnRNidec_enum)
  [VPMM_PowerSta_enum] -> "MCU_Rr Signal Error "/6(VPMM_PowerSta_enum)
  [No_CAN3_BUS_OFF] -> "MCU_Rr Signal Error "/5(No_CAN3_BUS_OFF)
  [VDDM_MCUNR1CSErrCFS_flg] -> "MCU_Rr Signal Error "/4(VDDM_MCUNR1CSErrCFS_flg)
  [VDDM_MCUNR1RCErrCFS_flg] -> "MCU_Rr Signal Error "/3(VDDM_MCUNR1RCErrCFS_flg)
  [VDDM_MCUNR1NoComCFS_flg] -> "MCU_Rr Signal Error "/2(VDDM_MCUNR1NoComCFS_flg)
  VINP_MCUWarnRNidec_enum/1 -> [VINP_MCUWarnRNidec_enum]
  VDDM_MCUNR1NoComCFS_flg/1 -> [VDDM_MCUNR1NoComCFS_flg]
  No_CAN3_BUS_OFF/1 -> [No_CAN3_BUS_OFF]
  VPMM_PowerSta_enum/1 -> [VPMM_PowerSta_enum]
  DTC_clear_request/1 -> [DTC_clear_request]
  "MCU_Rr Signal Error "/1(VDDM_RrMCUSigErrCFS_flg) -> [VDDM_RrMCUSigErrCFS_flg]
  [VDDM_RrMCUSigErrCFS_flg] -> VDDM_RrMCUSigErrCFS_flg/1
  VDDM_MCUNR1RCErrCFS_flg/1 -> [VDDM_MCUNR1RCErrCFS_flg]
  VDDM_MCUNR1CSErrCFS_flg/1 -> [VDDM_MCUNR1CSErrCFS_flg]

== system ddm/DDM/DDM/VMC_DDM/Shifter Signal Error ==
  task_time_s : Inport
  VDDM_Shifter1NoComCFS_flg : Inport  Port=2
  VDDM_Shifter1RCErrCFS_flg : Inport  Port=3
  VDDM_Shifter1CSErrCFS_flg : Inport  Port=4
  No_CAN3_BUS_OFF : Inport  Port=5
  VPMM_PowerSta_enum : Inport  Port=6
  VINP_ShifterFailsta_enum : Inport  Port=7
  DTC_clear_request : Inport  Port=8
  VTQD_GearActualPosn_enum : Inport  Port=9
  "Shifter Signal Error " : Subsystem
  VDDM_ShifterSigErrCFS_flg : Outport
  VDDM_ShifterSigErrDetDTC_raw32 : Outport  Port=2
  wires:
  [VTQD_GearActualPosn_enum] -> "Shifter Signal Error "/9(VTQD_GearActualPosn_enum)
  VTQD_GearActualPosn_enum/1 -> [VTQD_GearActualPosn_enum]
  [VDDM_ShifterSigErrDetDTC_raw32] -> VDDM_ShifterSigErrDetDTC_raw32/1
  "Shifter Signal Error "/2(VDDM_ShifterSigErrDetDTC_raw32) -> [VDDM_ShifterSigErrDetDTC_raw32]
  [task_time_s] -> "Shifter Signal Error "/1(task_time_s)
  task_time_s/1 -> [task_time_s]  "task_time_s"
  [DTC_clear_request] -> "Shifter Signal Error "/8(DTC_clear_request)
  [VINP_ShifterFailsta_enum] -> "Shifter Signal Error "/7(VINP_ShifterFailsta_enum)
  [VPMM_PowerSta_enum] -> "Shifter Signal Error "/6(VPMM_PowerSta_enum)
  [No_CAN3_BUS_OFF] -> "Shifter Signal Error "/5(No_CAN3_BUS_OFF)
  [VDDM_Shifter1CSErrCFS_flg] -> "Shifter Signal Error "/4(VDDM_Shifter1CSErrCFS_flg)
  [VDDM_Shifter1RCErrCFS_flg] -> "Shifter Signal Error "/3(VDDM_Shifter1RCErrCFS_flg)
  [VDDM_Shifter1NoComCFS_flg] -> "Shifter Signal Error "/2(VDDM_Shifter1NoComCFS_flg)
  VINP_ShifterFailsta_enum/1 -> [VINP_ShifterFailsta_enum]
  VDDM_Shifter1NoComCFS_flg/1 -> [VDDM_Shifter1NoComCFS_flg]
  No_CAN3_BUS_OFF/1 -> [No_CAN3_BUS_OFF]
  VPMM_PowerSta_enum/1 -> [VPMM_PowerSta_enum]
  DTC_clear_request/1 -> [DTC_clear_request]
  "Shifter Signal Error "/1(VDDM_ShifterSigErrCFS_flg) -> [VDDM_ShifterSigErrCFS_flg]
  [VDDM_ShifterSigErrCFS_flg] -> VDDM_ShifterSigErrCFS_flg/1
  VDDM_Shifter1RCErrCFS_flg/1 -> [VDDM_Shifter1RCErrCFS_flg]
  VDDM_Shifter1CSErrCFS_flg/1 -> [VDDM_Shifter1CSErrCFS_flg]

== system ddm/DDM/DDM/VMC_DDM/Zone_Dr_VCU ==
  note: Release Condiction After Decision
  note: Zone_Dr VCU Lost Comm (DrVCUNoCom)
  note: Diagnostics and Fault Handling
  task_time_s : Inport
  VPMM_PowerSta_enum : Inport  Port=2
  No_CAN4_BUS_OFF : Inport  Port=3
  VDDM_DrVCUNoCom_flg : Inport  Port=4
  DTC_clear_request : Inport  Port=5
  Constant : Constant  Value=ENUM_POWERSTA_OFF
  Constant1 : Constant  Value=ENUM_POWERSTA_OFF
  Constant10 : Constant  Value=FALSE
  Constant28 : Constant  Value=KDDM_DrVCUNoComDTC_cnt
  Constant29 : Constant  Value=KDDM_DrVCUNoComPassTO_s
  Constant30 : Constant  Value=KDDM_DrVCUNoComDetTO_s
  Constant4 : Constant  Value=KDDM_VMCDiagnosisOffSW_flg
  Constant49 : Constant  Value=ENUM_POWERSTA_OFF
  Constant5 : Constant  Value=ZERO_INT
  Constant52 : Constant  Value=ENUM_POWERSTA_STANDBY
  Constant55 : Constant  Value=KDDM_DrVCUNoComPassTO_s
  Constant9 : Constant  Value=KDDM_DrVCUNoComDTC_cnt
  DTC_Couter2 : hcu_lib/Basic_Blocks/DTC_Couter
  DTC_Info : hcu_lib/Basic_Blocks/DTC_Info
  Delay : Delay  DelayLength=1
  Equal : RelationalOperator  Operator=~=  OutDataTypeStr=boolean  RndMeth=Simplest
  Equal1 : RelationalOperator  Operator=~=  OutDataTypeStr=boolean  RndMeth=Simplest
  Equal20 : RelationalOperator  OutDataTypeStr=boolean  RndMeth=Simplest
  Equal3 : RelationalOperator  Operator===  OutDataTypeStr=boolean  RndMeth=Simplest
  Equal4 : RelationalOperator  Operator===  OutDataTypeStr=boolean  RndMeth=Simplest
  Logical Operator19 : Logic  Operator=NOT  AllPortsSameDT=off  OutDataTypeStr=boolean
  Logical Operator2 : Logic  AllPortsSameDT=off  OutDataTypeStr=boolean
  Logical Operator3 : Logic  Operator=OR  Inputs=4  AllPortsSameDT=off  OutDataTypeStr=boolean
  Logical Operator4 : Logic  Inputs=3  AllPortsSameDT=off  OutDataTypeStr=boolean
  Logical Operator50 : Logic  Inputs=3  AllPortsSameDT=off  OutDataTypeStr=boolean
  Logical Operator53 : Logic  Operator=NOT  AllPortsSameDT=off  OutDataTypeStr=boolean
  Logical Operator8 : Logic  AllPortsSameDT=off  OutDataTypeStr=boolean
  NOT : Logic  Operator=NOT  AllPortsSameDT=off  OutDataTypeStr=boolean
  Relational Operator : RelationalOperator  Operator=>  OutDataTypeStr=boolean  RndMeth=Simplest
  Switch5 : Switch  Criteria=u2 ~= 0
  Terminator : Terminator
  Test Detection Criteria2 : hcu_lib/Basic_Blocks/Test Detection Criteria
  Timer3 : hcu_lib/Basic_Blocks/Timer
  Unit Delay3 : UnitDelay  SampleTime=-1  HasFrameUpgradeWarning=on
  VDDM_DrVCUNoComCFS_flg : Outport
  VDDM_DrVCUNoComDTC_raw32 : Outport  Port=2
  wires:
  Switch5/1 -> Test Detection Criteria2/1
  Constant10/1 -> Switch5/1
  [VDDM_DrVCUNoComCFSRls_flg] -> Switch5/2
  [VDDM_DrVCUNoComDet_flg] -> DTC_Info/1
  [VDDM_DrVCUNoComPass_flg] -> DTC_Info/2
  [VDDM_DrVCUNoComCFS_flg] -> DTC_Info/3
  [DTC_clear_request] -> DTC_Info/4
  DTC_Info/1 -> [VDDM_DrVCUNoComDTC_raw32]  "VDDM_DrVCUNoComDTC_raw32"
  [VPMM_PowerSta_enum] -> Equal1/1
  Constant1/1 -> Equal1/2
  [VPMM_PowerSta_enum] -> Equal/1
  Constant/1 -> Equal/2
  [VDDM_DrVCUNoCom_flg] -> Logical Operator4/3
  [VDDM_DrVCUNoComCFS_flg] -> Delay/1
  Delay/1 -> NOT/1
  NOT/1 -> Logical Operator2/2
  Constant5/1 -> Relational Operator/2
  DTC_Couter2/1 -> [VDDM_DrVCUNoComCFS_flg]  "VDDM_DrVCUNoComCFS_flg"
  Constant4/1 -> Logical Operator3/4
  [VDDM_DrVCUNoComPass_flg] -> Logical Operator2/1
  Logical Operator2/1 -> Logical Operator3/3
  Equal20/1 -> [VDDM_DrVCUNoComPass_flg]  "VDDM_DrVCUNoComPass_flg"
  Constant52/1 -> Equal4/2
  Unit Delay3/1 -> Equal3/1
  Equal3/1 -> Logical Operator8/1
  Logical Operator4/1 -> Switch5/3
  [No_CAN4_BUS_OFF] -> Logical Operator50/2
  VDDM_DrVCUNoCom_flg/1 -> [VDDM_DrVCUNoCom_flg]
  [No_CAN4_BUS_OFF] -> Logical Operator4/2
  Logical Operator8/1 -> Logical Operator3/1
  Constant9/1 -> DTC_Couter2/3
  No_CAN4_BUS_OFF/1 -> [No_CAN4_BUS_OFF]
  Constant28/1 -> Test Detection Criteria2/3
  task_time_s/1 -> [task_time_s]
  [task_time_s] -> Timer3/3
  Logical Operator50/1 -> Logical Operator19/1, Timer3/1
  [task_time_s] -> Test Detection Criteria2/2
  Relational Operator/1 -> Terminator/1  "VDDM_DrVCUNoComDFS_flg"
  Logical Operator3/1 -> [VDDM_DrVCUNoComCFSRls_flg]  "VDDM_DrVCUNoComCFSRls_flg"
  Logical Operator53/1 -> Logical Operator50/3
  [VPMM_PowerSta_enum] -> Unit Delay3/1
  Equal4/1 -> Logical Operator8/2
  Constant29/1 -> Equal20/2
  DTC_clear_request/1 -> [DTC_clear_request]
  [DTC_clear_request] -> Logical Operator3/2
  Timer3/1 -> Equal20/1
  Logical Operator19/1 -> Timer3/2
  Test Detection Criteria2/1 -> [VDDM_DrVCUNoComDet_flg]  "VDDM_DrVCUNoComDet_flg"
  DTC_Couter2/2 -> Relational Operator/1  "VDDM_DrVCUNoComDTC_cnt"
  Constant49/1 -> Equal3/2
  VPMM_PowerSta_enum/1 -> [VPMM_PowerSta_enum]
  Constant55/1 -> Timer3/4
  [VDDM_DrVCUNoComDet_flg] -> DTC_Couter2/1
  Constant30/1 -> Test Detection Criteria2/4
  [VPMM_PowerSta_enum] -> Equal4/1
  [VDDM_DrVCUNoComCFSRls_flg] -> DTC_Couter2/2
  Equal/1 -> Logical Operator4/1
  Equal1/1 -> Logical Operator50/1
  [VDDM_DrVCUNoComDTC_raw32] -> VDDM_DrVCUNoComDTC_raw32/1
  [VDDM_DrVCUNoComCFS_flg] -> VDDM_DrVCUNoComCFS_flg/1
  [VDDM_DrVCUNoCom_flg] -> Logical Operator53/1
